simulink library "Lib_Vol_Pipe_TMATS_org"  (Simulink 10.0)
settings: Solver=ode45  StartTime=0.0  StopTime=10.0  RelTol=1e-3  EnableMultiTasking=on
undefined symbols (not defined in the file): Fluid
libraries: Lib_Vol_PropLookup_TMATS x3, simulink x1
Description:
  | Thomas Modules
settings Model: Creator=jwchapm2  LastModifiedBy=bhisma

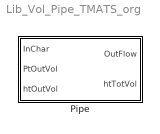
== system Lib_Vol_Pipe_TMATS_org ==
  Pipe : Subsystem  TreatAsAtomicUnit=on  mask(T-MATS: Pipe Library Block){Diameter=1, Length=24, htVec_M=Fluid.Vec.ht, PtVec_M=Fluid.Vec.Pt, TtArray_M=Fluid.Array.Tt, rhoArray_M=Fluid.Array.rho}
      mask prompts: Diameter "Diameter of pipe (in)"; Length "Length of pipe (in)"; htVec_M "htVec_M - Temperature Vector"; PtVec_M "PtVec_M - Pressure Vector"; TtArray_M "TtArray_M - Total Temperature Array f(ht,Pt)"; rhoArray_M "rhoArray_M - density f(ht,Pt)"
      mask help: This block simulates the performance of a duct using basic fluid dynamic equations and properties.
      mask Help: web(which('Vol_TMATS_pipe.html'),'-helpbrowser')

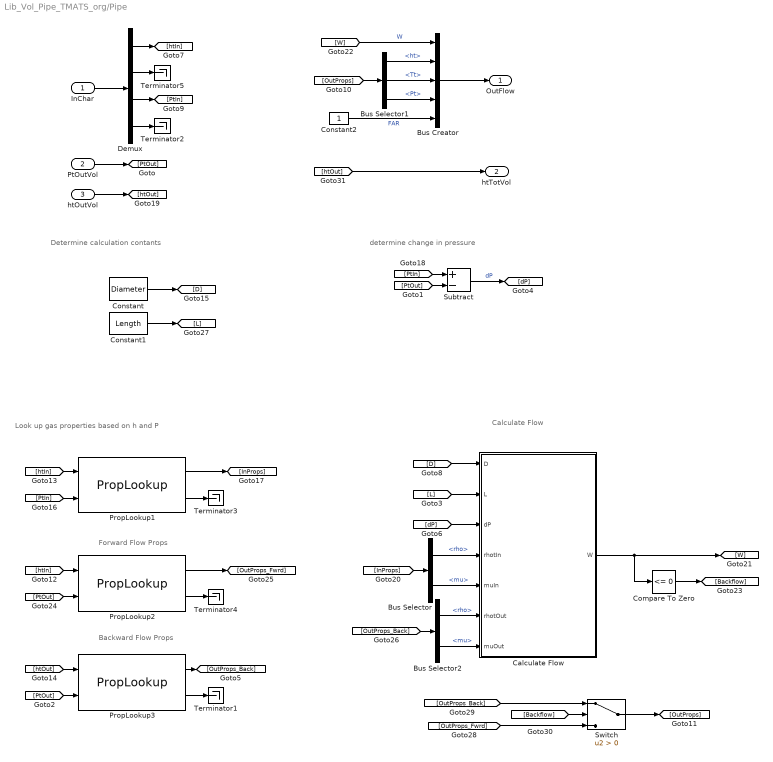
== system Lib_Vol_Pipe_TMATS_org/Pipe ==
  note: Look up gas properties based on h and P
  note: Calculate Flow
  note: Determine calculation contants
  note: determine change in pressure
  note: Backward Flow Props
  note: Forward Flow Props
  InChar : Inport
  PtOutVol : Inport  Port=2
  htOutVol : Inport  Port=3
  Bus Creator : BusCreator  Inputs=5
  Bus Selector : BusSelector  OutputSignals=rho,mu
  Bus Selector1 : BusSelector  OutputSignals=ht,Tt,Pt
  Bus Selector2 : BusSelector  OutputSignals=rho,mu
  Calculate Flow : MATLAB Function  TreatAsAtomicUnit=on
  Compare To Zero : simulink/Logic and Bit Operations/Compare To Zero  relop=<=  OutDataTypeStr=boolean
  Constant : Constant  Value=Diameter
  Constant1 : Constant  Value=Length
  Constant2 : Constant
  Demux : Demux
  PropLookup1 : Lib_Vol_PropLookup_TMATS/PropLookup  case_M='ht'  propg_M=0  htg_M=0  htVec_M=htVec_M  PtVec_M=PtVec_M  TtVec_M=[-10000 10000]  sVec_M=[-10000 10000]  htArray_M=ones(2, length(PtVec_M))'  rhoArray_M=rhoArray_M  uArray_M=ones(length(htVec_M), length(PtVec_M))'  sArray_M=ones(length(htVec_M), length(PtVec_M))'  muArray_M=ones(length(htVec_M), length(PtVec_M))'  ThArray_M=TtArray_M  CvArray_M=ones(length(htVec_M), length(PtVec_M))'  CpArray_M=ones(length(htVec_M), length(PtVec_M))'  kArray_M=ones(length(htVec_M), length(PtVec_M))'  TsArray_M=ones(2, length(PtVec_M))'  hsArray_M=ones(2, length(PtVec_M))'  Rval_M=0
  PropLookup2 : Lib_Vol_PropLookup_TMATS/PropLookup  case_M='ht'  propg_M=0  htg_M=0  htVec_M=htVec_M  PtVec_M=PtVec_M  TtVec_M=[-10000 10000]  sVec_M=[-10000 10000]  htArray_M=ones(2, length(PtVec_M))'  rhoArray_M=rhoArray_M  uArray_M=ones(length(htVec_M), length(PtVec_M))'  sArray_M=ones(length(htVec_M), length(PtVec_M))'  muArray_M=ones(length(htVec_M), length(PtVec_M))'  ThArray_M=TtArray_M  CvArray_M=ones(length(htVec_M), length(PtVec_M))'  CpArray_M=ones(length(htVec_M), length(PtVec_M))'  kArray_M=ones(length(htVec_M), length(PtVec_M))'  TsArray_M=ones(2, length(PtVec_M))'  hsArray_M=ones(2, length(PtVec_M))'  Rval_M=0
  PropLookup3 : Lib_Vol_PropLookup_TMATS/PropLookup  case_M='ht'  propg_M=0  htg_M=0  htVec_M=htVec_M  PtVec_M=PtVec_M  TtVec_M=[-10000 10000]  sVec_M=[-10000 10000]  htArray_M=ones(2, length(PtVec_M))'  rhoArray_M=rhoArray_M  uArray_M=ones(length(htVec_M), length(PtVec_M))'  sArray_M=ones(length(htVec_M), length(PtVec_M))'  muArray_M=ones(length(htVec_M), length(PtVec_M))'  ThArray_M=TtArray_M  CvArray_M=ones(length(htVec_M), length(PtVec_M))'  CpArray_M=ones(length(htVec_M), length(PtVec_M))'  kArray_M=ones(length(htVec_M), length(PtVec_M))'  TsArray_M=ones(2, length(PtVec_M))'  hsArray_M=ones(2, length(PtVec_M))'  Rval_M=0
  Subtract : Sum  Inputs=+-
  Switch : Switch  Criteria=u2 > Threshold
  Terminator{1..5} (5 alike) : Terminator
  OutFlow : Outport  PortDimensions=5
  htTotVol : Outport  Port=2  PortDimensions=1
  wires:
  Constant1/1 -> [L]
  [L] -> Calculate Flow/2(L)
  Bus Selector2/2 -> Calculate Flow/7(muOut)  "<mu>"
  Bus Selector/2 -> Calculate Flow/5(muIn)  "<mu>"
  Constant/1 -> [D]
  Subtract/1 -> [dP]  "dP"
  PropLookup3/1 -> [OutProps_Back]
  PropLookup3/2 -> Terminator1/1
  PtOutVol/1 -> [PtOut]
  [PtOut] -> Subtract/2
  [PtOut] -> PropLookup3/2
  [htOut] -> PropLookup3/1
  [PtIn] -> Subtract/1
  htOutVol/1 -> [htOut]
  [D] -> Calculate Flow/1(D)
  [dP] -> Calculate Flow/3(dP)
  InChar/1 -> Demux/1
  Demux/1 -> [htIn]
  Demux/4 -> Terminator2/1
  Demux/3 -> [PtIn]
  Demux/2 -> Terminator5/1
  PropLookup1/1 -> [InProps]
  PropLookup1/2 -> Terminator3/1
  [PtIn] -> PropLookup1/2
  [htIn] -> PropLookup1/1
  [InProps] -> Bus Selector/1
  Bus Selector/1 -> Calculate Flow/4(rhotIn)  "<rho>"
  [W] -> Bus Creator/1  "W"
  [OutProps] -> Bus Selector1/1
  Bus Selector1/1 -> Bus Creator/2  "<ht>"
  Bus Selector1/2 -> Bus Creator/3  "<Tt>"
  Bus Selector1/3 -> Bus Creator/4  "<Pt>"
  Constant2/1 -> Bus Creator/5  "FAR"
  Bus Creator/1 -> OutFlow/1
  [htOut] -> htTotVol/1
  Calculate Flow/1(W) -> [W], Compare To Zero/1
  Compare To Zero/1 -> [Backflow]
  Switch/1 -> [OutProps]
  [OutProps_Back] -> Switch/1
  [OutProps_Fwrd] -> Switch/3
  [Backflow] -> Switch/2
  PropLookup2/1 -> [OutProps_Fwrd]
  PropLookup2/2 -> Terminator4/1
  [PtOut] -> PropLookup2/2
  [htIn] -> PropLookup2/1
  Bus Selector2/1 -> Calculate Flow/6(rhotOut)  "<rho>"
  [OutProps_Back] -> Bus Selector2/1

== matlab function Pipe/Calculate Flow ==
  data: D input double; L input double; W output double; dP input double; rhotIn input double; muIn input double; rhotOut input double; muOut input double
function W = fcn(D,L,dP,rhotIn,muIn,rhotOut,muOut)
%#codegen
%Fully developed laminar and turbulent mass flow rates are calculated based
%on mean velocity for cirular cross section pipes. Reynolds number are then
%calculated to determine the appropriate mass flow rate i.e. Reynolds
%numbers greater than 2000 are assumed turbulent. 
if dP > 0
      W_lam = dP*(rhotIn/12/12/12)*pi*(D/2)^4/(8*muIn*L);
      W_tur = rhotIn/12/12/12*((dP*D^4.75)/(0.242*L*muIn^0.25*(rhotIn/12/12/12)^0.75))^(1/1.75);
      R_lam = 2*W_lam/(pi*D/2*muIn);
%       R_tur = 2*W_tur/(pi*D/2*muIn);
      if R_lam > 2000
          W = W_tur;
      else
          W = W_lam;
      end
else
      W_lam = -dP*(rhotOut/12/12/12)*pi*(D/2)^4/(8*muOut*L);
      W_tur = -rhotOut/12/12/12*((-dP*D^4.75)/(0.242*L*muOut^0.25*(rhotOut/12/12/12)^0.75))^(1/1.75);
      R_lam = 2*W_lam/(pi*D/2*muOut);
%       R_tur = 2*W_tur/(pi*D/2*muOut);
      if R_lam > 2000
          W = W_tur;
      else
          W = W_lam;
      end
end
